simulink model "slexMaskDrawingExamples"  (R2022b)
settings: Solver=FixedStepDiscrete  StartTime=0.0  StopTime=10.0  FixedStep=1  RelTol=1e-3  EnableMultiTasking=on
PreLoadFcn:
  | addpath(fullfile(matlabroot,'examples','simulink_masking','main'));
Description:
  | slexMaskDrawingExamples
  | 
  | This example highlights various features of mask icon.
settings Model: Creator=The MathWorks, Inc.  LastModifiedBy=The MathWorks, Inc.
settings SolverCC: AlgebraicLoopSolver=TrustRegion  MaxZcPerStep=1
settings DataIOCC: LimitDataPoints=on  SaveFormat=Array  ReturnWorkspaceOutputs=off
settings OptimizationCC: ExpressionDepthLimit=2147483647  LifeSpan=inf
settings DebuggingCC: UnderspecifiedInitializationDetection=Classic  MergeDetectMultiDrivingBlocksExec=none  SolverPrmCheckMsg=warning  UnconnectedInputMsg=warning  UnconnectedOutputMsg=warning  UnconnectedLineMsg=warning  AllowSymbolicDim=off  StateNameClashWarn=warning  SFUnexpectedBacktrackingDiag=warning  SFNoUnconditionalDefaultTransitionDiag=warning  SFExecutionAtInitializationDiag=none  SFMachineParentedDataDiag=warning  ArithmeticOperatorsInVariantConditions=warning
settings HardwareCC: ProdBitPerPointer=32  ProdBitPerSizeT=32  ProdBitPerPtrDiffT=32  ProdLargestAtomicFloat=None  ProdIntDivRoundTo=Undefined  ProdEndianess=Unspecified  ProdWordSize=32  ProdHWDeviceType=32-bit Generic
settings ModelReferenceCC: EnableRefExpFcnMdlSchedulingChecks=on  PropagateSignalLabelsOutOfModel=off
settings SFSimCC: SimUseLocalCustomCode=off  CustomCodeUndefinedFunction=UseInterfaceOnly
settings RTWCC: RTWUseLocalCustomCode=off  DLArmComputeVersion=19.05
settings CodeAppCC: StateflowObjectComments=on
settings GRTTargetCC: TargetLangStandard=C89/C90 (ANSI)
settings ConfigComp: CovMetricSettings=dw  CovSaveCumulativeToWorkspaceVar=on  CovSaveSingleToWorkspaceVar=on  CovExternalEMLEnable=off

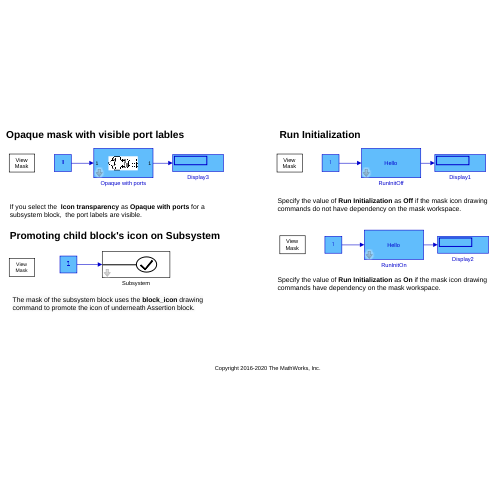
[thumbnail: Simulink's stored preview of the top-level diagram]
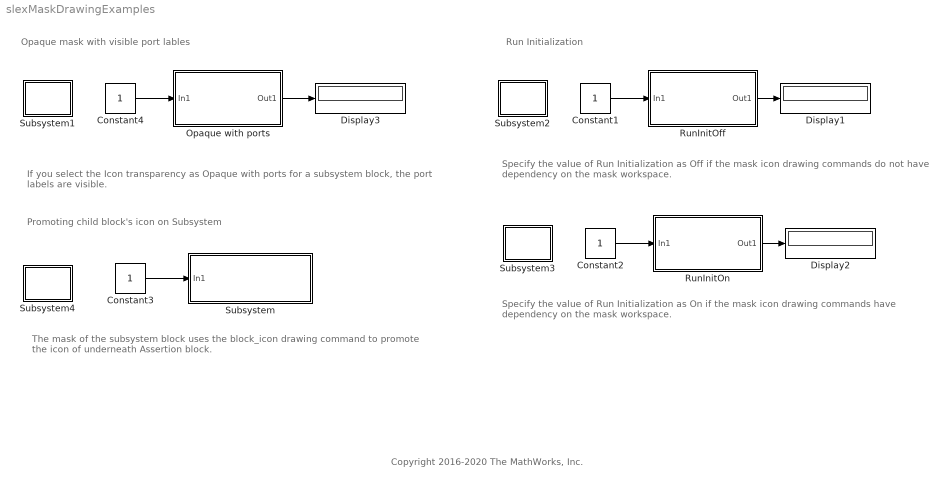
== system slexMaskDrawingExamples ==
  note: Specify the value of Run Initialization as Off if the mask icon drawing commands do not have dependency on the mask workspace.
  note: Run Initialization
  note: If you select the Icon transparency as Opaque with ports for a subsystem block, the port labels are visible.
  note: Opaque mask with visible port lables
  note: Copyright 2016-2020 The MathWorks, Inc.
  note: Specify the value of Run Initialization as On if the mask icon drawing commands have dependency on the mask workspace.
  note: The mask of the subsystem block uses the block_icon drawing command to promote the icon of underneath Assertion block.
  note: Promoting child block's icon on Subsystem
  Constant{1..4} (4 alike) : Constant
  Display1 : Display
  Display2 : Display
  Display3 : Display
  Opaque with ports : Subsystem
      settings: DeleteFcn=slexUtilityCloseMaskExample(get_param(gcb, 'handle'));
      mask Display: image('aeropropulsion1.bmp','center')
  RunInitOff : Subsystem  mask{Parameter1=343434, Parameter2=45345454}
      mask prompts: Parameter1 "Input Value"; Parameter2 "Ouput Value"
      settings: DeleteFcn=slexUtilityCloseMaskExample(get_param(gcb, 'handle'));
      mask Display: disp('Hello')
  RunInitOn : Subsystem  mask{parameter1='Hello'}
      mask prompts: parameter1 "Specify mask icon value"
      settings: DeleteFcn=slexUtilityCloseMaskExample(get_param(gcb, 'handle'));
      mask Display: disp(parameter1)
  Subsystem : Subsystem  mask{Parameter1=0}
      mask Display: block_icon('Assertion')
  Subsystem1 : Subsystem
      settings: OpenFcn=slexUtilityOpenMaskTabExample(get_param([gcs, '/Opaque with ports'], 'handle'), 0);
      mask Display: disp('View\nMask')
  Subsystem2 : Subsystem
      settings: OpenFcn=slexUtilityOpenMaskTabExample(get_param([gcs, '/RunInitOff'], 'handle'), 0);
      mask Display: disp('View\nMask')
  Subsystem3 : Subsystem
      settings: OpenFcn=slexUtilityOpenMaskTabExample(get_param([gcs, '/RunInitOn'], 'handle'), 0);
      mask Display: disp('View\nMask')
  Subsystem4 : Subsystem
      settings: OpenFcn=slexUtilityOpenMaskTabExample(get_param([gcs, '/Subsystem'], 'handle'), 0);
      mask Display: disp('View\nMask')
  wires:
  Constant2/1 -> RunInitOn/1(In1)
  RunInitOff/1(Out1) -> Display1/1
  Constant1/1 -> RunInitOff/1(In1)
  Opaque with ports/1(Out1) -> Display3/1
  Constant4/1 -> Opaque with ports/1(In1)
  RunInitOn/1(Out1) -> Display2/1
  Constant3/1 -> Subsystem/1(In1)

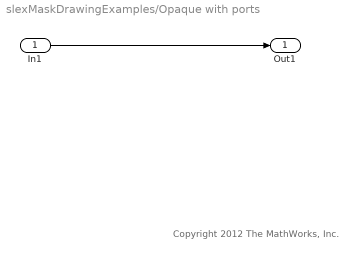
== system slexMaskDrawingExamples/Opaque with ports ==
  note: Copyright 2012 The MathWorks, Inc.
  In1 : Inport
  Out1 : Outport  VectorParamsAs1DForOutWhenUnconnected=off
  wires:
  In1/1 -> Out1/1

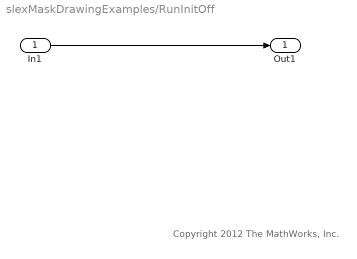
== system slexMaskDrawingExamples/RunInitOff ==
  note: Copyright 2012 The MathWorks, Inc.
  In1 : Inport
  Out1 : Outport  VectorParamsAs1DForOutWhenUnconnected=off
  wires:
  In1/1 -> Out1/1

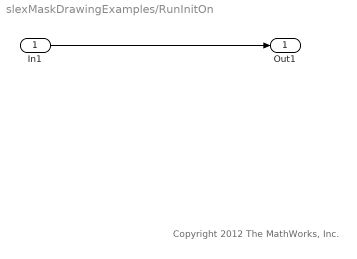
== system slexMaskDrawingExamples/RunInitOn ==
  note: Copyright 2012 The MathWorks, Inc.
  In1 : Inport
  Out1 : Outport  VectorParamsAs1DForOutWhenUnconnected=off
  wires:
  In1/1 -> Out1/1

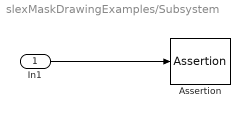
== system slexMaskDrawingExamples/Subsystem ==
  In1 : Inport
  Assertion : Assertion
  wires:
  In1/1 -> Assertion/1

== system slexMaskDrawingExamples/Subsystem1 ==

== system slexMaskDrawingExamples/Subsystem2 ==

== system slexMaskDrawingExamples/Subsystem3 ==

== system slexMaskDrawingExamples/Subsystem4 ==
